simulink model "clab_3_2_sim"  (R2014a)
settings: Solver=ode45  StartTime=0.0  StopTime=5  RelTol=1e-3
values from neighbouring files (symbols this model uses):
  alpha = 7600    [clab3_1.m]    (also in clab3_2.m)
  beta = 2000    [clab3_1.m]    (also in clab3_2.m = 1430)
  C = 15000    [clab3_2.m]
  lambda = 2470    [clab3_2.m]
  mu = 7200    [clab3_1.m]    (also in clab3_2.m)
  phi = 0.51    [clab3_1.m]    (also in clab3_2.m)
  Ql = 8400    [clab3_1.m]    (also in clab3_2.m)
  theta = 2.5    [clab3_1.m]    (also in clab3_2.m)
  v = 139000    [clab3_1.m]    (also in clab3_2.m = 70000)
settings Model: Creator=Tommy  LastModifiedBy=Tommy

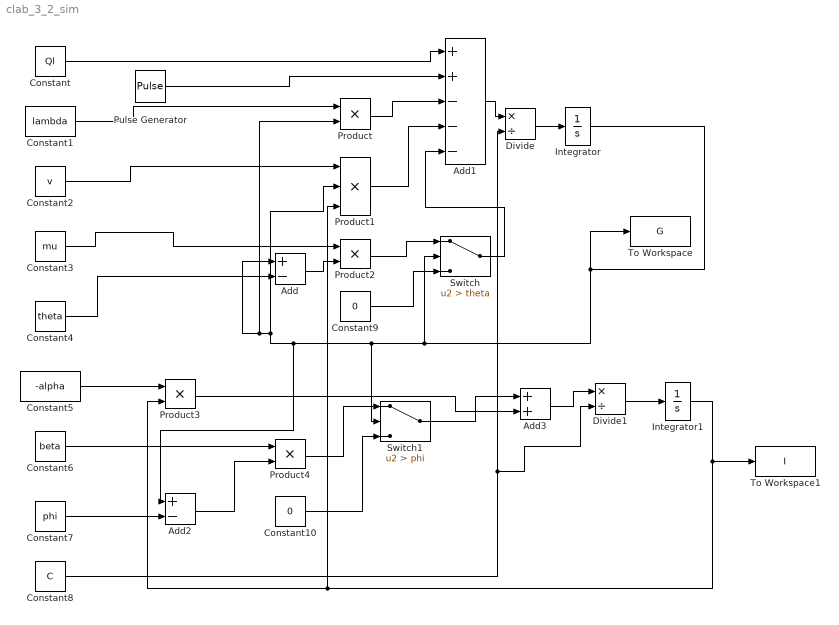
== system clab_3_2_sim ==
  Add : Sum  Inputs=+-
  Add1 : Sum  Inputs=++---
  Add2 : Sum  Inputs=+-
  Add3 : Sum
  Constant : Constant  Value=Ql
  Constant1 : Constant  Value=lambda
  Constant10 : Constant  Value=0
  Constant2 : Constant  Value=v
  Constant3 : Constant  Value=mu
  Constant4 : Constant  Value=theta
  Constant5 : Constant  Value=-alpha
  Constant6 : Constant  Value=beta
  Constant7 : Constant  Value=phi
  Constant8 : Constant  Value=C
  Constant9 : Constant  Value=0
  Divide : Product  Inputs=*/
  Divide1 : Product  Inputs=*/
  Integrator : Integrator
  Integrator1 : Integrator
  Product{,2..4} (4 alike) : Product
  Product1 : Product  Inputs=3
  Pulse Generator : DiscretePulseGenerator  PulseType=Time based  Amplitude=100000  Period=5  PulseWidth=5  PhaseDelay=.5
  Switch : Switch  Criteria=u2 > Threshold  Threshold=theta
  Switch1 : Switch  Criteria=u2 > Threshold  Threshold=phi
  To Workspace : ToWorkspace  VariableName=G  SaveFormat=Timeseries  SampleTime=-1
  To Workspace1 : ToWorkspace  VariableName=I  SaveFormat=Timeseries  SampleTime=-1
  wires:
  Constant/1 -> Add1/1
  Constant1/1 -> Product/1
  Constant2/1 -> Product1/1
  Product/1 -> Add1/3
  Product1/1 -> Add1/4
  Constant4/1 -> Add/2
  Add/1 -> Product2/2
  Constant3/1 -> Product2/1
  Integrator/1 -> To Workspace/1, Switch/2, Switch1/2, Add2/1, Product1/2, Product/2, Add/1
  Switch/1 -> Add1/5
  Product2/1 -> Switch/1
  Constant9/1 -> Switch/3
  Add1/1 -> Divide/1
  Divide/1 -> Integrator/1
  Constant8/1 -> Divide1/2, Divide/2
  Constant5/1 -> Product3/1
  Constant6/1 -> Product4/1
  Constant7/1 -> Add2/2
  Add2/1 -> Product4/2
  Product4/1 -> Switch1/1
  Constant10/1 -> Switch1/3
  Switch1/1 -> Add3/1
  Product3/1 -> Add3/2
  Add3/1 -> Divide1/1
  Divide1/1 -> Integrator1/1
  Integrator1/1 -> Product1/3, Product3/2, To Workspace1/1
  Pulse Generator/1 -> Add1/2
